simulink model "testee"  (R2022b)
settings: Solver=VariableStepAuto  StartTime=0.0  StopTime=30  RelTol=1e-3
values from neighbouring files (symbols this model uses):
  Cd = [0 1.092]    [lab11.m]    (also in lab13.m)
  F = [0.001 -0.382; 0.35 0.739]    [lab11.m]    (also in lab13.m)
  H = [0.35; 0.239]    [lab11.m]    (also in lab13.m)
  kd1 = acker(F, H, jd1)    [teste.m]
  T = 0.5    [teste.m]
undefined symbols (not defined in the file or in its folder): kd2
settings Model: Creator=hugo_  LastModifiedBy=hugo_

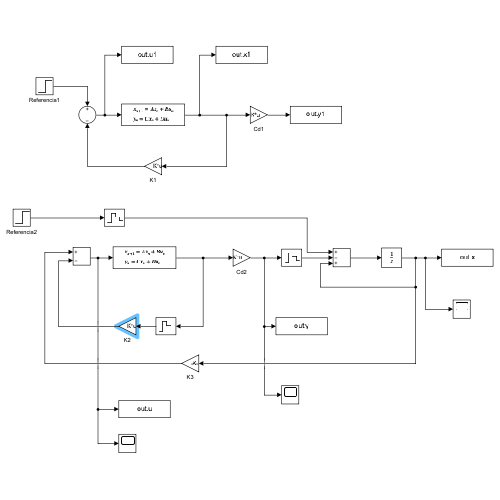
[thumbnail: Simulink's stored preview of the top-level diagram]
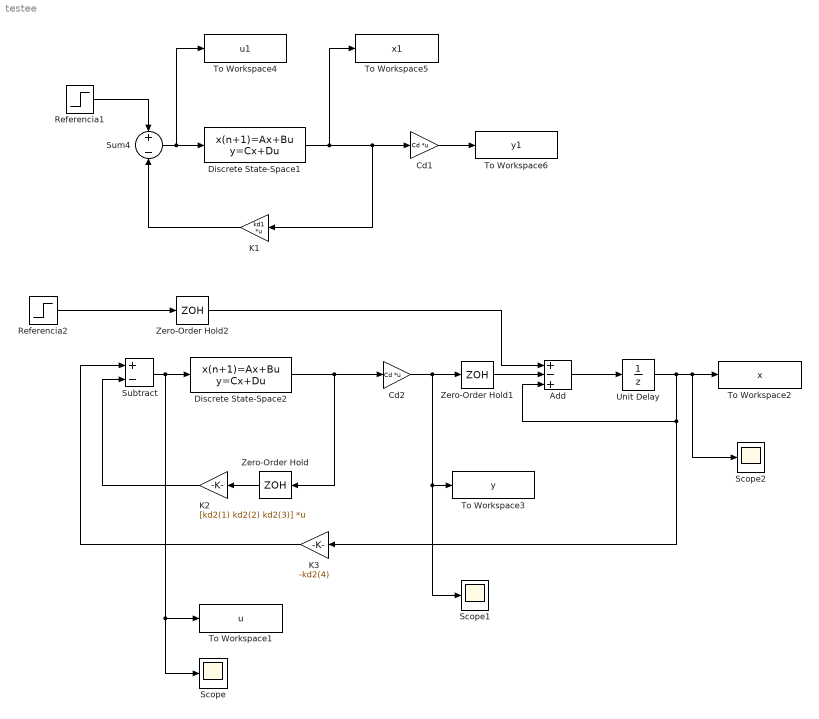
== system testee ==
  Add : Sum  Inputs=+-+
  Cd1 : Gain  Gain=Cd  Multiplication=Matrix(K*u)
  Cd2 : Gain  Gain=Cd  Multiplication=Matrix(K*u)
  Discrete State-Space1 : DiscreteStateSpace  A=F  B=H  C=[1 0 0; 0 1 0; 0 0 1]  D=[0;0;0]  SampleTime=T
  Discrete State-Space2 : DiscreteStateSpace  A=F  B=H  C=[1 0 0; 0 1 0; 0 0 1]  D=[0;0;0]  SampleTime=T
  K1 : Gain  Gain=kd1  Multiplication=Matrix(K*u)
  K2 : Gain  Gain=[kd2(1) kd2(2) kd2(3)]  Multiplication=Matrix(K*u)
  K3 : Gain  Gain=-kd2(4)
  Referencia1 : Step  Time=0  SampleTime=0
  Referencia2 : Step  Time=0  SampleTime=0
  Scope : Scope
  Scope1 : Scope
  Scope2 : Scope
  Subtract : Sum  Inputs=+-
  Sum4 : Sum  Inputs=+|-
  To Workspace1 : ToWorkspace  VariableName=u  SaveFormat=Timeseries  SampleTime=-1
  To Workspace2 : ToWorkspace  VariableName=x  SaveFormat=Timeseries  SampleTime=-1
  To Workspace3 : ToWorkspace  VariableName=y  SaveFormat=Timeseries  SampleTime=-1
  To Workspace4 : ToWorkspace  VariableName=u1  SaveFormat=Timeseries  SampleTime=-1
  To Workspace5 : ToWorkspace  VariableName=x1  SaveFormat=Timeseries  SampleTime=-1
  To Workspace6 : ToWorkspace  VariableName=y1  SaveFormat=Timeseries  SampleTime=-1
  Unit Delay : UnitDelay  SampleTime=-1  HasFrameUpgradeWarning=on
  Zero-Order Hold : ZeroOrderHold  SampleTime=T
  Zero-Order Hold1 : ZeroOrderHold  SampleTime=T
  Zero-Order Hold2 : ZeroOrderHold  SampleTime=T
  wires:
  Cd1/1 -> To Workspace6/1
  Referencia1/1 -> Sum4/1
  Sum4/1 -> To Workspace4/1, Discrete State-Space1/1
  Discrete State-Space1/1 -> To Workspace5/1, K1/1, Cd1/1
  K1/1 -> Sum4/2
  Discrete State-Space2/1 -> Zero-Order Hold/1, Cd2/1
  Zero-Order Hold/1 -> K2/1
  K2/1 -> Subtract/2
  Subtract/1 -> Scope/1, To Workspace1/1, Discrete State-Space2/1
  Cd2/1 -> Scope1/1, To Workspace3/1, Zero-Order Hold1/1
  Zero-Order Hold1/1 -> Add/2
  Referencia2/1 -> Zero-Order Hold2/1
  Zero-Order Hold2/1 -> Add/1
  Add/1 -> Unit Delay/1
  Unit Delay/1 -> Scope2/1, To Workspace2/1, K3/1, Add/3
  K3/1 -> Subtract/1
